simulink model "VFlexP_small"  (R2026a)
settings: Solver=ode23tb  StopTime=2  FixedStep=5e-5
values from neighbouring files (symbols this model uses):
  block_idx = evalin(mdlWks, [bvarname Generators{i} '_idx'])    [fun_init_units_callback.m]
  Fb = areas    [fun_MATPOWER_to_Excel.m]
  Fi = evalin('base', get_param(block, 'Fi'))    [fun_init_GFr.m]    (also in fun_init_intconv_DC_VSM.m)
  Lf = evalin('base', get_param(block, 'Lf'))    [fun_init_GFr.m]    (also in fun_init_intconv_DC_VSM.m)
  Rf = evalin('base', get_param(block, 'Rf'))    [fun_init_GFr.m]    (also in fun_init_intconv_DC_VSM.m)
symbols that are objects in the model workspace (value not decoded): Grid_DCop_DC_PES, Grid_DCop_DCBUCK, Grid_op_CCVSC, Grid_op_IG, Grid_op_SG, Grid_op_VSM, Grid_opDC_CCVSC, Grid_opDC_VSM, Grid_opGFr, Grid_opVCVSC
undefined symbols (not defined in the file or in its folder): block_buses_DC, CCVSC_idx, Cf, costs, costs2, DFIGs_nodes, DiscIntNeverNeededParam, entity, From_nodes, grid_linsys, Grid_op_DFIG, Grid_op_DFIG_PQ, Grid_op_MSG, Grid_op_SC, Grid_op_VCVSC, Hv, initial_states_grid, Kic, Kiv, Kp_theta, Kp_w, Kpc, Kpv, last_send, Lc, m, Matrix_flux_to_i, mD, mp, MSGs_buses, Nbuses_DC, nq, op_VCVSC, Psche, Rc, rkq1, rkq2, SCs_buses, SCs_nodes, sec_control_structure, set_asked, set_DG_up, set_extra_satur, set_sending_cost, SGs_buses, SGs_nodes, Tf, To_nodes, VI_L, VI_R, WOF_Tf, xkq1, xkq2
libraries: simulink x1045, eeGeneralControl x12, eeTransforms x1, sl_discontinuities x1
(part 1 of 50)
settings Model: Creator=atomas  LastModifiedBy=atomas
settings SolverCC: ZeroCrossControl=DisableAll
settings DataIOCC: InitialState=getstatestruct(op1)  SaveFormat=StructureWithTime
settings DebuggingCC: ReadBeforeWriteMsg=DisableAll  WriteAfterWriteMsg=DisableAll  WriteAfterReadMsg=DisableAll  MultiTaskDSMMsg=none  UnderSpecifiedDimensionMsg=warning
settings SFSimCC: SFSimEcho=off
settings SimscapeCC: SimscapeNominalValues="[{\"value\":\"1\",\"unit\":\"A\"},{\"value\":\"1\",\"unit\":\"bar\"},{\"value\":\"1\",\"unit\":\"cm^2\"},{\"value\":\"1\",\"unit\":\"cm^3/s\"},{\"value\":\"1\",\"unit\":\"kJ/kg\"},{\"value\":\"1\",\"unit\":\"kW\"},{\"value\":\"1\",\"unit\":\"l\"},{\"value\":\"1\",\"unit\":\"N\"},{\"value\":\"1\",\"unit\":\"N*m\"},{\"value\":\"1\",\"unit\":\"V\"}]"  SimscapeLogType=none  SimscapeLogDataHistory=5000.0

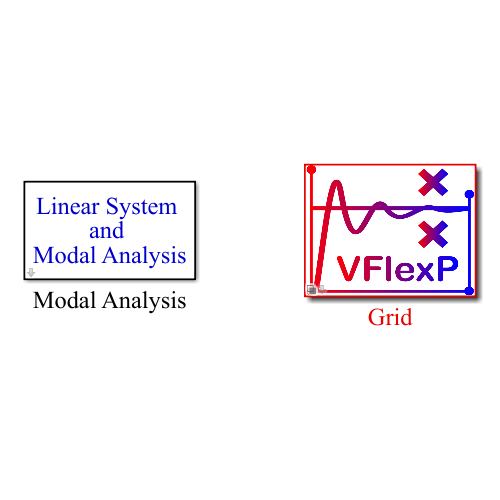
[thumbnail: Simulink's stored preview of the top-level diagram]
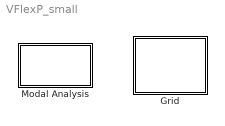
== system VFlexP_small ==
  Grid : Subsystem  Variant=on  VariantControlMode=label  VariantControl=Choice  LabelModeActiveChoice=Dynamic  mask(Grid){bvarname=Grid_, Sb=0.015, Fb_data={ '1', '50' }, bus_data={ '1', '3', '0.005', '0', '0.0001', '0.0001', '1', '1.0000000000', '0.0000000000', '230', '1', '1.1', '0.9', 'dynamic', 'series RL static omega', 'dynamic', 'PQ'; '2', '1', '0.005', '0', '0.0001', '0.0001', '1', '1.0000000000', '-0.0435875362', '230', '1', '1.1', '0.9', 'dynamic', 'series RL static omega', 'dynamic', 'PQ'; '3', '1', '0', '0', '0.0001', '0', '2', '1.0000000000', '0.6174487396', '230', '1', '1.1', '0.9', 'DC dynamic', 'DC ConstR', 'dynamic', 'PQ' }, gen_data={ '1', 'GFr', '0.0053259727', '-0.0001225105', '1000', '-1000', '1', '100', '1', '1000', '-100', '0', '0', '0', '0', '0', '0', '0', '0', '0', '0', '0'; '3', 'DC_PES', '0.0050000000', '0.0000000000', '1000', '-1000', '1', '100', '1', '1000', '-100', '0', '0', '0', '0', '0', '0', '0', '0', '0', '0', '0' }, line_data={ '1', '2', '0.005', '0.05', '0', '0', '0', '0', '0', '0', '1', '-360', '360', 'dynamic', 'static omega' }, save_in_workspace=off, parameter_change_filename=1, param_change_data={}, SC_structure=No SC, define_SC_in_MATLAB=on, delayM=0, passM=1, A_f_sc=1, A_P_sc=1, A_v_sc=1, A_Q_sc=1, g_f_sc=1, g_P_sc=1, g_v_sc=1, g_Q_sc=1, intconv_data={ 'DC_VSM', '3', '2', '0.0003', '0.0355', '0', '1000', '1000', '1000', '1', '0', '1', '-360', '360', '0', '0', '0', '0', '0', '0', '0', '0', '1', '1', '1.22', '0.75', '1', '0', '1', '-0.5', '0.5', '-360', '360', '0', '0.001', '0.0015', '0.002', '0' }, TC_structure=No TC}
      mask prompts: Sb "Base power (MW)"; Fb_data "Base frequency (Hz)"; save_in_workspace "Save in Workspace"; parameter_change_filename "Filename "Parameter_Change_V_""; SC_structure "Secondary control structure"; define_SC_in_MATLAB "Define control structure in MATLAB"; TC_structure "Tertiary control structure"
      mask init:
      | bvarname = [matlab.lang.makeValidName(get_param(gcb, 'Name')) '_'];
      |     set_param(gcb, "bvarname", bvarname)
      |     mdlWks = get_param(bdroot,'ModelWorkspace'); % Get the model workspace
      | 
      |     % Initialise variables
      |     v_buses_mod = [];
      |     Cbuses = [];
      |     DGs = [];
      |     From_buses = [];
      |     L_Lines = [];
      |     shift_lines = [];
      |     tap_lines = [];
      |     L_Loads = [];
      |     Load_buses = [];
      |     Nbuses = [];
      |     PQ_gen = [];
      |     Ploads = [];
      |     Ps_lf = [];
      |     Qloads = [];
      |     Qs_lf = [];
      |     R_Lines = [];
      |     C_Lines = [];
      |     R_Loads = [];
      |     Rcf = [];
      |     To_buses = [];
      |     Lines_fromM = [];
      |     Lines_toM = [];
      |     iPs_lf = [];
      |     iQs_lf = [];
      |     bus = [];
      |     buses_lf = [];
      |     line_complexity = [];
      |     bus_complexity = [];
      |     load_complexity = [];
      |     line_complexity_PF = [];
      |     bus_complexity_PF = [];
      |     load_complexity_PF = [];
      |     admitt_matrix = [];
      |     iadmitt_matrix = [];
      |     admitt_matrix_noloads = [];
      |     iadmitt_matrix_noloads = [];
      |     gen_static_params = [];
      |     gen_to_plot = 1;
      |     loadDC_complexity = [];
      |     lineDC_complexity = [];
      |     busDC_complexity = [];
      |     loadDC_complexity_PF = [];
      |     lineDC_complexity_PF = [];
      |     busDC_complexity_PF = [];
      |     fref.ref_units = 1;
      |     omega_base = 2*pi*50;
      | 
      |     bl = find_system([gcb '/Dynamic/Generators'], ...
      |         'IncludeCommented', 'on', 'SearchDepth', '2', ...
      |         'LookUnderMasks', 'on', 'Name', 'trim_output');
      |     for i = 1:length(bl) 
      |        DG_namei = get_param(get_param(bl{i}, 'Parent'), 'Name');
      |        eval([DG_namei 's = [];']);
      |        eval([DG_namei 's_buses = 1;']);
      |        eval([DG_namei '_idx = [];']);
      |     end
      | 
      |     try
      |         v_buses_mod = mdlWks.getVariable([bvarname 'v_buses_mod']);
      |         Cbuses = mdlWks.getVariable([bvarname 'Cbuses']);
      |         DGs = mdlWks.getVariable([bvarname 'DGs']);
      |         gen_static_params = mdlWks.getVariable([bvarname 'gen_static_params']);
      |         From_buses = mdlWks.getVariable([bvarname 'From_buses']);
      |         L_Lines = mdlWks.getVariable([bvarname 'L_Lines']);
      |         tap_lines = mdlWks.getVariable([bvarname 'tap_lines']);
      |         shift_lines = mdlWks.getVariable([bvarname 'shift_lines']);
      |         L_Loads = mdlWks.getVariable([bvarname 'L_Loads']);
      |         Load_buses = mdlWks.getVariable([bvarname 'Load_buses']);
      |         Load_busesDC = mdlWks.getVariable([bvarname 'Load_busesDC']);
      |         Nbuses = mdlWks.getVariable([bvarname 'Nbuses']);
      |         PQ_gen = mdlWks.getVariable([bvarname 'PQ_gen']);
      |         Ploads = mdlWks.getVariable([bvarname 'Ploads']);
      |         Ps_lf = mdlWks.getVariable([bvarname 'Ps_lf']);
      |         Qloads = mdlWks.getVariable([bvarname 'Qloads']);
      |         Qs_lf = mdlWks.getVariable([bvarname 'Qs_lf']);
      |         R_Lines = mdlWks.getVariable([bvarname 'R_Lines']);
      |         C_Lines = mdlWks.getVariable([bvarname 'C_Lines']);
      |         R_Loads = mdlWks.getVariable([bvarname 'R_Loads']);
      |         Rcf = mdlWks.getVariable([bvarname 'Rcf']);
      |         To_buses = mdlWks.getVariable([bvarname 'To_buses']);
      |         Lines_fromM = mdlWks.getVariable([bvarname 'Lines_fromM']);
      |         Lines_toM = mdlWks.getVariable([bvarname 'Lines_toM']);
      |         iPs_lf = mdlWks.getVariable([bvarname 'iPs_lf']);
      |         iQs_lf = mdlWks.getVariable([bvarname 'iQs_lf']);
      |         bus = mdlWks.getVariable([bvarname 'bus']);
      |         buses_lf = mdlWks.getVariable([bvarname 'buses_lf']);
      |         PloadsDC = mdlWks.getVariable([bvarname 'PloadsDC']);
      |         R_Loads_DC = mdlWks.getVariable([bvarname 'R_Loads_DC']);
      |         line_complexity = mdlWks.getVariable([bvarname 'line_complexity']);
      |         bus_complexity = mdlWks.getVariable([bvarname 'bus_complexity']);
      |         load_complexity = mdlWks.getVariable([bvarname 'load_complexity']);
      |         line_complexity_PF = mdlWks.getVariable([bvarname 'line_complexity_PF']);
      |         bus_complexity_PF = mdlWks.getVariable([bvarname 'bus_complexity_PF']);
      |         load_complexity_PF = mdlWks.getVariable([bvarname 'load_complexity_PF']);
      |         admitt_matrix = mdlWks.getVariable([bvarname 'admitt_matrix']);
      |         iadmitt_matrix = mdlWks.getVariable([bvarname 'iadmitt_matrix']);
      |         admitt_matrix_noloads = mdlWks.getVariable([bvarname 'admitt_matrix_noloads']);
      |         iadmitt_matrix_noloads = mdlWks.getVariable([bvarname 'iadmitt_matrix_noloads']);
      |         conductance_matrix = mdlWks.getVariable([bvarname 'conductance_matrix']);
      |         iconductance_matrix = mdlWks.getVariable([bvarname 'iconductance_matrix']);
      |         conductance_matrix_noloads = mdlWks.getVariable([bvarname 'conductance_matrix_noloads']);
      |         iconductance_matrix_noloads = mdlWks.getVariable([bvarname 'iconductance_matrix_noloads']);
      |         loadDC_complexity = mdlWks.getVariable([bvarname 'loadDC_complexity']);
      |         loadDC_complexity_PF = mdlWks.getVariable([bvarname 'loadDC_complexity_PF']);
      |         lineDC_complexity = mdlWks.getVariable([bvarname 'lineDC_complexity']);
      |         lineDC_complexity_PF = mdlWks.getVariable([bvarname 'lineDC_complexity_PF']);
      |         busDC_complexity = mdlWks.getVariable([bvarname 'busDC_complexity']);
      |         busDC_complexity_PF = mdlWks.getVariable([bvarname 'busDC_complexity_PF']);
      |         
      |         
      |         if length(buses_lf) <= 25
      |             gen_to_plot = 1:length(buses_lf);
      |         end
      |         for i = 1:length(bl)
      |            try
      |                DG_namei = get_param(get_param(bl{i}, 'Parent'), 'Name');
      |                aux1 = mdlWks.getVariable([bvarname DG_namei 's']);
      |                aux2 = mdlWks.getVariable([bvarname DG_namei 's_buses']);
      |                aux4 = mdlWks.getVariable([bvarname DG_namei '_idx']);
      |                eval([DG_namei 's = aux1;']);
      |                eval([DG_namei 's_buses = aux2;']);
      |                eval([DG_namei '_idx = aux4;']);
      |            catch
      |            end
      |         end
      |     if strcmp(get_param(gcb, "LabelModeActiveChoice"), "Dynamic") ...
      |                 && (strcmp(get_param([gcb '/Dynamic/Secondary Control'], ...
      |                 "LabelModeActiveChoice"), "Matrices")...
      |                 || strcmp(get_param([gcb '/Dynamic/Secondary Control'], ...
      |                 "LabelModeActiveChoice"), "Matrices1")...
      |                 || strcmp(get_param([gcb '/Dynamic/Secondary Control'], ...
      |                 "LabelModeActiveChoice"), "Matrices with delay")) ...
      |                 && ~define_SC_in_MATLAB
      |         DGs_number = length(buses_lf);
      |         delayM = 0.1*circshift(eye(DGs_number), 1);
      |         passM = circshift(eye(DGs_number), 1);
      |         A_f_sc = circshift(eye(DGs_number), 1);
      |         A_P_sc = circshift(eye(DGs_number), 1);
      |         A_v_sc = eye(DGs_number);
      |         A_Q_sc = circshift(eye(DGs_number), 1);
      |         A_f_sc(1,:) = 0;
      |         A_P_sc(1,:) = 0;
      |         A_v_sc(1,:) = 0;
      |         A_Q_sc(1,:) = 0;
      |         A_f_sc(1,1) = 0; % Leader follows reference frequency
      |         A_P_sc(1,1) = 1; % Leader is slack
      |         A_Q_sc(1,1) = 1; % Leader is slack
      |         g_f_sc = zeros(1, DGs_number);
      |         g_P_sc = zeros(1, DGs_number);
      |         g_v_sc = zeros(1, DGs_number);
      |         g_Q_sc = zeros(1, DGs_number);
      |         g_f_sc(1) = 1; % Leader follows reference frequency
      |         g_v_sc(1) = 1; % Leader follows reference voltage
      |     elseif strcmp(get_param(gcb, "LabelModeActiveChoice"), "Dynamic") ...
      |                 && strcmp(get_param([gcb '/Dynamic/Secondary Control'], ...
      |                 "LabelModeActiveChoice"), ...
      |                 "Matrices with delay and limitation") && ~define_SC_in_MATLAB
      |         DGs_number = length(buses_lf);
      |         delayM = 0*0.1*circshift(eye(DGs_number), 1);
      |         passM = circshift(eye(DGs_number), 1);
      |         A_f_sc = circshift(eye(DGs_number), 1);
      |         A_P_sc = circshift(eye(DGs_number), 1);
      |         A_v_sc = circshift(eye(DGs_number), 1);
      |         A_Q_sc = circshift(eye(DGs_number), 1);
      |         g_f_sc = zeros(1, DGs_number);
      |         g_P_sc = zeros(1, DGs_number);
      |         g_v_sc = zeros(1, DGs_number);
      |         g_Q_sc = zeros(1, DGs_number);
      |         g_f_sc(1) = 1; % Leader follows reference frequency
      |         g_v_sc(1) = 1; % Leader follows reference voltage
      |     end
      | 
      |     catch ME
      |         %errordlg(ME.message)
      |     end
      |     try
      |         DC = mdlWks.getVariable([bvarname 'DC']);
      |         intconv_PF = mdlWks.getVariable([bvarname 'intconv_PF']);
      |         fref = mdlWks.getVariable([bvarname 'fref']);
      |         omega_base = 2*pi*cell2mat(Fb_data(:,2))';
      |     catch ME
      |         %errordlg(ME.message)
      |     end
      mask Help: web('doc_Home.html')
      mask Callback bus_data: fun_bus_data_callback(gcb)
      mask Callback gen_data: fun_gen_data_callback(gcb)
      mask Callback line_data: fun_line_data_callback(gcb)
      mask Callback param_change_data: fun_apply_changes_block(gcb)
      mask TypeOptions SC_structure: No SC | Pilot nodes | Matrices | Matrices1 | Matrices with delay | Matrices with delay and limitation | MAS UC | MAS UC binary | MAS messages
      mask Callback SC_structure:
      | set_param([gcb '/Dynamic/Secondary Control'],...
      |     'LabelModeActiveChoice', ...
      |     get_param(gcb, "SC_structure"))
      mask Callback define_SC_in_MATLAB:
      | p = Simulink.Mask.get(gcb); param = p.getDialogControl('tSC_table');
      | if strcmp(get_param(gcb, "define_SC_in_MATLAB"), 'off')
      |     param.Visible = 'off';
      | else
      |     param.Visible = 'on';
      | end
      mask Callback intconv_data: fun_intconv_data_callback(gcb)
      mask TypeOptions TC_structure: No TC | MAS edp | MAS messages | Scheduled
      mask Callback TC_structure:
      | set_param([gcb '/Dynamic/Tertiary Control'],...
      |     'LabelModeActiveChoice', ...
      |     get_param(gcb, "TC_structure"))
      mask DialogControl load_system Prompt: Load system
      mask DialogControl load_system Callback: fun_load_system_callback(gcb)
      mask DialogControl save_table Prompt: Save table file
      mask DialogControl save_table Callback: fun_save_table_callback(gcb)
      mask DialogControl MATPOWER_loadflow Prompt: MATPOWER Loadflow
      mask DialogControl MATPOWER_loadflow Callback: fun_MATPOWER_loadflow(gcb)
      mask DialogControl loadflow Prompt: Loadflow
      mask DialogControl loadflow Callback: fun_loadflow_callback(gcb)
      mask DialogControl lf_report Prompt: Loadflow report
      mask DialogControl lf_report Callback: fun_lf_report_callback(gcb)
      mask DialogControl init_units Prompt: Initialise units
      mask DialogControl init_units Callback: fun_init_units_callback(gcb)
      mask DialogControl load_complexity Prompt: Load complexity in grid
      mask DialogControl load_complexity Callback: fun_load_complexity_grid(gcb)
      mask DialogControl Scope_gen Prompt: Show generators signals
      mask DialogControl Scope_gen Callback: open_system([gcb '/Dynamic/Scope_gen'])
      mask DialogControl simulate_simulink Prompt: Simulate
      mask DialogControl simulate_simulink Callback:
      | model = bdroot;
      | sim(model);
      mask DialogControl Control34 Prompt: Instituto de Investigación Tecnológica. <br> Universidad Pontificia Comillas.
      mask DialogControl Control34 Callback: web('https://www.iit.comillas.edu/')
      mask DialogControl home_tab Prompt: System parameters
      mask DialogControl new_row_Fb Prompt: +
      mask DialogControl new_row_Fb Callback: fun_mask_new_row_Fb(gcb)
      mask DialogControl delete_row_Fb Prompt: -
      mask DialogControl delete_row_Fb Callback: fun_mask_delete_row_Fb(gcb)
      mask DialogControl clear_Fb_table Prompt: Clear
      mask DialogControl clear_Fb_table Callback:
      | maskObj = Simulink.Mask.get(gcb);
      |     tableControl = maskObj.getDialogControl( 'Fb_data' );
      |     for i=1:tableControl.getNumberOfRows()
      |         tableControl.removeRow(1);
      |     end
      mask DialogControl bus_tab Prompt: Bus data
      mask DialogControl new_row_bus Prompt: +
      mask DialogControl new_row_bus Callback: fun_mask_new_row_Bus(gcb)
      mask DialogControl delete_row_bus Prompt: -
      mask DialogControl delete_row_bus Callback: fun_mask_delete_row_Bus(gcb)
      mask DialogControl clear_bus_table Prompt: Clear
      mask DialogControl clear_bus_table Callback:
      | maskObj = Simulink.Mask.get(gcb);
      |     tableControl = maskObj.getDialogControl( 'bus_data' );
      |     for i=1:tableControl.getNumberOfRows()
      |         tableControl.removeRow(1);
      |     end
      mask DialogControl gen_tab Prompt: Gen data
      mask DialogControl refresh_DGs Prompt: Refresh DG options
      mask DialogControl refresh_DGs Callback: fun_refresh_DGs_callback(gcb)
      mask DialogControl open_DG Prompt: Open DGs configuration
      mask DialogControl open_DG Callback: fun_open_DG_callback(gcb)
      mask DialogControl new_row_gen Prompt: +
      mask DialogControl new_row_gen Callback: fun_mask_new_row_Gen(gcb)
      mask DialogControl delete_row_gen Prompt: -
      mask DialogControl delete_row_gen Callback: fun_mask_delete_row_Gen(gcb)
      mask DialogControl clear_gen_table Prompt: Clear
      mask DialogControl clear_gen_table Callback:
      | maskObj = Simulink.Mask.get(gcb);
      |     tableControl = maskObj.getDialogControl( 'gen_data' );
      |     for i=1:tableControl.getNumberOfRows()
      |         tableControl.removeRow(1);
      |     end
      mask DialogControl line_tab Prompt: Line data
      mask DialogControl new_row_line Prompt: +
      mask DialogControl new_row_line Callback: fun_mask_new_row_Line(gcb)
      mask DialogControl delete_row_line Prompt: -
      mask DialogControl delete_row_line Callback: fun_mask_delete_row_Line(gcb)
      mask DialogControl clear_line_table Prompt: Clear
      mask DialogControl clear_line_table Callback:
      | maskObj = Simulink.Mask.get(gcb);
      |     tableControl = maskObj.getDialogControl( 'line_data' );
      |     for i=1:tableControl.getNumberOfRows()
      |         tableControl.removeRow(1);
      |     end
      mask DialogControl param_change Prompt: Parameter Variation
      mask DialogControl execute_parameter_change Prompt: Execute Parameter Change
      mask DialogControl execute_parameter_change Callback: fun_execute_parameter_change(gcb)
      mask DialogControl new_parameter Prompt: +
      mask DialogControl new_parameter Callback: fun_mask_new_row_Param(gcb)
      mask DialogControl delete_parameter Prompt: -
      mask DialogControl delete_parameter Callback: fun_mask_delete_row_Param(gcb)
      mask DialogControl clear_param_table Prompt: Clear
      mask DialogControl clear_param_table Callback:
      | maskObj = Simulink.Mask.get(gcb);
      |     tableControl = maskObj.getDialogControl( 'param_change_data' );
      |     for i=1:tableControl.getNumberOfRows()
      |         tableControl.removeRow(1);
      |     end
      mask DialogControl plot_change_parameter Prompt: Plot Selected Parameter
      mask DialogControl plot_change_parameter Callback: fun_plot_change_parameter_callback(gcb)
      mask DialogControl Secondary_control Prompt: Secondary control
      mask DialogControl Construct_MAS Prompt: Construct_MAS
      mask DialogControl Construct_MAS Callback: fun_construct_MAS_callback(gcb)
      mask DialogControl Initialise_0 Prompt: Initialise all variables to 0
      mask DialogControl Initialise_0 Callback: fun_initialise_0_callback(gcb)
      mask DialogControl intconv_tab Prompt: Int converters
      mask DialogControl new_row_intconv Prompt: +
      mask DialogControl new_row_intconv Callback: fun_mask_new_row_Intconv(gcb)
      mask DialogControl delete_row_intconv Prompt: -
      mask DialogControl delete_row_intconv Callback: fun_mask_delete_row_Intconv(gcb)
      mask DialogControl clear_intconv_tabl Prompt: Clear
      mask DialogControl clear_intconv_tabl Callback:
      | maskObj = Simulink.Mask.get(gcb);
      |     tableControl = maskObj.getDialogControl( 'intconv_data' );
      |     for i=1:tableControl.getNumberOfRows()
      |         tableControl.removeRow(1);
      |     end
      mask DialogControl Tertiary_control Prompt: Tertiary control
      mask DialogControl Construct_MAS_tertiary Prompt: Construct_MAS
      mask DialogControl Construct_MAS_tertiary Callback: fun_construct_MAS_callback(gcb)
      mask DialogControl Initialise_0_copy Prompt: Initialise all variables to 0
      mask DialogControl Initialise_0_copy Callback: fun_initialise_0_callback(gcb)
      mask Display: image('$imagefile');
  Modal Analysis : Subsystem
      mask Help: web([extractBefore(get_param(bdroot, 'FileName'), ['\' gcs '.slx']) '\Documentation\modal_analysis.html'])
      mask DialogControl DescTextVar Prompt: FAST MODAL ANALYSIS TOOL
      mask DialogControl ParameterGroupVar Prompt: ANALYSIS
      mask DialogControl calculate_linsys Prompt: Calculate Linear System
      mask DialogControl calculate_linsys Callback:
      | wb = waitbar(0, 'Linearizing the system', 'Name','Linear System Option'); % Waitbar
      |     model = bdroot;
      |     io = getlinio(model);
      |     waitbar(0.25,wb)
      |     try
      |         linsys = linearize(model,io);
      |          waitbar(0.5,wb)
      |         if height(linsys)>1
      |             linsys = linsys(1,1);
      |         end
      |             waitbar(0.75,wb)
      |         modelworkspace=get_param(model,"ModelWorkspace");
      | 
      |         assignin("base","linsys",linsys);
      |         assignin(modelworkspace,"linsys",linsys);
      |         waitbar(1,wb)
      | 
      |     catch
      |         try
      |         waitbar(0.5,wb)
      |         linsys = linearize(model,io);
      |         waitbar(0.75,wb)
      |         if height(linsys)>1
      |             linsys = linsys(1,1);
      |         end
      |         waitbar(1,wb)
      |         modelworkspace=get_param(model,"ModelWorkspace");
      | 
      |         assignin("base","linsys",linsys);
      |         assignin(modelworkspace,"linsys",linsys);
      |         catch ME
      |              msg = ["There has being a problem calculating the modal analysis",...
      |             "Please check:"," - (1) you are working on the simulink model folder",...
      |             " - (2) The scripts for the linearized trigonometric functions are " + ...
      |             "in the same folder",...
      |             " - (3) There is still one input perturbation and one output measurement in the system"];
      |             errordlg(msg);
      |             errordlg(ME.message);
      |         end
      |     end
      | 
      |     close(wb)
      mask DialogControl modal_analysis_calculation Prompt: Modal Analysis Excel Generator
      mask DialogControl modal_analysis_calculation Callback:
      | wb = waitbar(0, 'Modal Analisys', 'Name','Exporting Modal Analysis Caculation'); % Waitbar
      | 
      |     model = bdroot;
      |     waitbar(0.25,wb)
      |     modelworkspace=get_param(model,"ModelWorkspace");
      |     linsys = evalin(modelworkspace,"linsys");
      |   if ~isempty(linsys)
      |         A = linsys.a;
      |       [v,z] = eig(A);
      |         n = height(A);
      |         % Eigenvalues
      |         z = diag(z) ;
      |         %[magz,iz]=sort(1./abs(z));
      |         [~,iz]=sort(1./imag(z));
      |         z = z(iz);
      |         v = v(:,iz);
      |         % Right eigenvectors
      |         for i = 1:n
      |           [~,imax] = max(abs(v(:,i))) ;
      |           v(:,i) = v(:,i)/v(imax,i) ;
      |         end
      |         % Left eigenvectors
      |         w=inv(v);
      |         % Participations
      |         for i = 1:n
      |           for j = 1:n
      |             p(i,j) = w(j,i)*v(i,j);
      |           end
      |         end
      |                 Xvec_vars = linsys.StateName;
      | 
      |     waitbar(0.5,wb)
      | 
      |     N = height(A);
      |     nombrevar = char(Xvec_vars);
      | 
      |     Variables_Names = char(nombrevar);
      |     Modes = string(1:N)';
      |     T1 = table(Variables_Names);
      |     T =  array2table(abs(p));
      |     T.Properties.VariableNames = Modes;
      |     TPart = [T1 T];
      |     waitbar(0.6,wb)
      | 
      |     TeigenvaluesTitle = ({'Eigenvalue'; 'REAL';'IMAGINARY';'DAMPING';'FREQUENCY'});
      |     Eig_Table = [ array2table([ (1:length(z))' real(z) imag(z) -real(z)./abs(z)*100,abs(z)./2/pi])];
      |     Eig_Table.Properties.VariableNames = TeigenvaluesTitle;
      |     waitbar(0.7,wb)
      | 
      |     unstable_eigenvalues = find(real(z)>0);
      | 
      |      if unstable_eigenvalues>1
      |         TPart_Unstable = sortrows([T1 TPart(:,unstable_eigenvalues+1)],2,{'descend'});
      |      end
      |     else
      |         msg = "There has being a problem calculating the modal analysis";
      |         f = warndlg(msg);
      |     end
      |     try
      |         filename ="ModalAnalysisTables.xlsx";
      |         writetable(sortrows(Eig_Table,4,{'ascend'}),filename,"Sheet","SUMMARY BY DAMPING");
      |         writetable(sortrows(Eig_Table,5,{'ascend'}),filename,"Sheet","SUMMARY BY FREQUENCY");
      |     waitbar(0.8,wb)
      | 
      |         writetable(TPart,filename,"Sheet","Participations");
      |         if (unstable_eigenvalues)>1
      |             writetable(TPart_Unstable,filename,"Sheet","Unstable Participations");
      |         else
      |             writematrix([0 0],filename,"Sheet","Unstable Participations");
      |         end
      |         writematrix([real(v) imag(v)],filename,"Sheet","Left Eigenvectors");
      |         waitbar(0.9,wb)
      | 
      |         writematrix([real(w) imag(w)],filename,"Sheet","Right Eigenvectors");
      |         waitbar(1,wb)
      | 
      |         msg = "TABLES HAVE BEEN CORRECTLY EXPORTED";
      |         f = warndlg(msg);
      |     catch
      |          msg = ["TABLES COULD NOT BE MADE"," MAKE SURE THE EXCEL IS CLOSED"];
      |          f = warndlg(msg);
      | 
      | 
      |     end
      |         close(wb)
      mask DialogControl plot_eigenvalues Prompt: Plot EigenValues
      mask DialogControl plot_eigenvalues Callback:
      | model = bdroot;
      | 
      |     modelworkspace=get_param(model,"ModelWorkspace");
      |     linsys = evalin(modelworkspace,"linsys");
      | 
      |     figure(1);clf;
      |     plot(real(eig(linsys.a)),imag(eig(linsys.a)),'*');
      |     grid on
      mask DialogControl plot_eigenvalues_mod_angle Prompt: Plot Eigenvalues Mod&Angle
      mask DialogControl plot_eigenvalues_mod_angle Callback:
      | model = bdroot;
      | 
      | modelworkspace=get_param(model,"ModelWorkspace");
      | linsys = evalin(modelworkspace,"linsys");
      | figure(1);clf;
      | loglog(abs(eig(linsys.a)),rad2deg(wrapTo2Pi(angle(eig(linsys.a)))),'*');
      | 
      | xlimit = log10(xlim); %ylimit = ylim;
      | 
      | for i=logspace(2*xlimit(1)-xlimit(2),xlimit(2),40)
      |     line(min(max(i./abs(cos(deg2rad(90:1:270))),0.99*10^xlimit(1)), ...
      |     1.01*10^xlimit(2)),90:1:270,'LineStyle','-','Color','black','HandleVisibility','off');
      | end
      | 
      | ylim([90-20 180])
      mask DialogControl run_andres_tool Prompt: Advanced Simulink Modal Analysis Tool
      mask DialogControl run_andres_tool Callback: simulink_modal_analysis(bdroot);
      mask DialogControl Container3 Prompt: CLEAR SYSTEMS
      mask DialogControl clear_simulink Prompt: Clear SIMULINK Workspace
      mask DialogControl clear_simulink Callback:
      | model = bdroot;
      |     command_clear = "clear all";
      | 
      |     modelworkspace=get_param(model,"ModelWorkspace");
      |     evalin(modelworkspace,command_clear)
      mask DialogControl clear_matlab Prompt: Clear MATLAB Workspaces
      mask DialogControl clear_matlab Callback:
      | command_clear = "clear all";
      |     evalin("base",command_clear)
      mask Display:
      | color('BLUE');
      | 
      | fprintf('Linear System \nand \nModal Analysis');

== system VFlexP_small/Grid ==
  Dynamic : Subsystem  VariantControl=Dynamic
  Loadflow : Subsystem  VariantControl=Loadflow

== system VFlexP_small/Modal Analysis ==

== system VFlexP_small/Grid/Dynamic ==
  Constant2 : Constant  Value=omega_base  VectorParams1D=off
  DCAC converters : Subsystem
  Display : Display
  Display1 : Display
  Display2 : Display
  Fault : Subsystem  Commented=on
  Gain : Gain  Gain=1/(2*pi)
  Gain1 : Gain  Gain=Sb
  Gain2 : Gain  Gain=Sb
  Gain3 : Gain  Gain=Sb
  Gain4 : Gain  Gain=0.5
  Gain{5..8} (4 alike) : Gain  Gain=50
  Generators : Subsystem
  Generators_DC : Subsystem
  Goto Tag Visibility : GotoTagVisibility  GotoTag=omega_ref
  Goto Tag Visibility1 : GotoTagVisibility  GotoTag=omega_base
  Grid : Subsystem  Variant=on  VariantControlMode=label  LabelModeActiveChoice=Dynamic
  Grid_DC : Subsystem  Variant=on  VariantControlMode=label  LabelModeActiveChoice=Dynamic
  Grid_linear : Subsystem  Commented=on
  Integrator : Integrator  InitialConditionSource=external
  Integrator1 : Integrator  InitialConditionSource=external
  LPF : Subsystem
  LPF1 : Subsystem
  LPF2 : Subsystem
  LPF3 : Subsystem
  Manual Switch : ManualSwitch
  One : Constant  OutDataTypeStr=Inherit: Inherit via back propagation
  Product1 : Product
  Product2 : Product
  Real-Imag to Complex1 : RealImagToComplex
  Real-Imag to Complex2 : RealImagToComplex
  Scope{,2..4} (4 alike) : Scope
      Scope settings: ActiveDisplayYMinimum=0.0022712  ActiveDisplayYMaximum=0.0044108
      Scope2 settings: ActiveDisplayYMinimum=49.851  ActiveDisplayYMaximum=50.0166  DataLoggingVariableName=ScopeData11
      Scope3 settings: ActiveDisplayYMinimum=49.8343  ActiveDisplayYMaximum=50.0185  DataLoggingVariableName=ScopeData12
      Scope4 settings: ActiveDisplayYMinimum=49.83966644890701  ActiveDisplayYMaximum=50.01785268343977
  Scope1 : Scope  NumInputPorts=2
      settings: ActiveDisplayYMinimum=-0.03276  ActiveDisplayYMaximum=0.28873  DataLoggingVariableName=ScopeData8
  Scope_gen : Scope  NumInputPorts=4
      settings: Title=Frequency (Hz)  ActiveDisplayYMinimum=49.889931736775623  ActiveDisplayYMaximum=50.01222980702493  DataLoggingVariableName=gen
  Secondary Control : Subsystem  Variant=on  VariantControlMode=label  VariantControl=Choice  LabelModeActiveChoice=No SC
      settings: PortSchema="{\"entries\":[{\"content\":{\"sides\":[{\"content\":{\"connectorIds\":[\"Out1\"]},\"type\":\"ConnectorPlacement.EquallySpacedRectSide\",\"uuid\":\"fff1731e-03ae-4532-8327-8c877d5503a1\"},{\"content\":{\"connectorIds\":[\"In1\",\"In2\",\"In3\",\"In4\"],\"side\":\"RIGHT\"},\"type\":\"ConnectorPlacement.EquallySpacedRectSide\",\"uuid\":\"a483b49e-8899-40e0-871c-863b08e1ecd3\"},{\"content\":{\"connectorIds\":[],\"side\":\"TOP\"},\"type\":\"ConnectorPlacement.EquallySpacedRectSide\",\"uuid\":\"d6acdfc2-068d-45c3-a7db-011142f68adc\"},{\"content\":{\"connectorIds\":[],\"side\":\"BOTTOM\"},\"type\":\"ConnectorPlacement.EquallySpacedRectSide\",\"uuid\":\"a007924e-be31-4ab9-87dc-62addce8969f\"}]},\"type\":\"ConnectorPlacement.EquallySpacedConnector\",\"uuid\":\"f40773b4-1769-44e6-aa19-3b4c4e232e75\"}],\"packageUris\":[\"http://schema.mathworks.com/mf0/Connector/R2020b\"],\"version\":\"1.0\"}"
  Selector : Selector  NumberOfDimensions=2  InputPortWidth=3  IndexOptions=Index vector (dialog),Index vector (dialog)  Indices=1,fref.ref_units  OutputSizes=1,1
  Selector1 : Selector  NumberOfDimensions=2  InputPortWidth=3  IndexOptions=Select all,Index vector (dialog)  Indices=[1 3],gen_to_plot  OutputSizes=1,1
  Selector10 : Selector  NumberOfDimensions=2  InputPortWidth=3  IndexOptions=Index vector (dialog),Select all  Indices=2,1  OutputSizes=1,1
  Selector11 : Selector  NumberOfDimensions=2  InputPortWidth=3  IndexOptions=Index vector (dialog),Select all  Indices=4,1  OutputSizes=1,1
  Selector2 : Selector  NumberOfDimensions=2  InputPortWidth=3  IndexOptions=Index vector (dialog),Index vector (dialog)  Indices=2,1  OutputSizes=1,1
  Selector3 : Selector  NumberOfDimensions=2  InputPortWidth=3  IndexOptions=Index vector (dialog),Select all  Indices=2,1  OutputSizes=1,1
  Selector4 : Selector  NumberOfDimensions=2  InputPortWidth=3  IndexOptions=Index vector (dialog),Index vector (dialog)  Indices=1,1  OutputSizes=1,1
  Selector5 : Selector  NumberOfDimensions=2  InputPortWidth=3  IndexOptions=Index vector (dialog),Select all  Indices=3,1  OutputSizes=1,1
  Selector7 : Selector  NumberOfDimensions=2  InputPortWidth=3  IndexOptions=Index vector (dialog),Select all  Indices=1,1  OutputSizes=1,1
  Selector8 : Selector  InputPortWidth=length(fref.ref_units)  IndexOptions=Index vector (dialog)  Indices=fref.Fb_units  OutputSizes=1
  Selector9 : Selector  NumberOfDimensions=2  InputPortWidth=3  IndexOptions=Index vector (dialog),Select all  Indices=1,1  OutputSizes=1,1
  Step : Step  Time=20  SampleTime=0  VectorParams1D=off  ZeroCross=off
  Step1 : Step  Time=10  InitialValue=ones(1, length(buses_lf))  FinalValue=[ones(1, length(buses_lf)-1) 1]  SampleTime=0  VectorParams1D=off  ZeroCross=off
  Subsystem1 : Subsystem  Commented=on
  Sum : Sum  Inputs=+++++
  Sum1 : Sum  Inputs=|++
  Sum2 : Sum  Inputs=|++
  Sum3 : Sum  Inputs=|+-
  Sum4 : Sum  Inputs=|+-
  Sum5 : Sum  Inputs=|++
  Terminator : Terminator
  Terminator1 : Terminator
  Tertiary Control : Subsystem  Variant=on  VariantControlMode=label  VariantControl=Choice  LabelModeActiveChoice=No TC
      settings: PortSchema="{\"entries\":[{\"content\":{\"sides\":[{\"content\":{\"connectorIds\":[\"Out1\"]},\"type\":\"ConnectorPlacement.EquallySpacedRectSide\",\"uuid\":\"fff1731e-03ae-4532-8327-8c877d5503a1\"},{\"content\":{\"connectorIds\":[\"In1\",\"In2\",\"In3\"],\"side\":\"RIGHT\"},\"type\":\"ConnectorPlacement.EquallySpacedRectSide\",\"uuid\":\"a483b49e-8899-40e0-871c-863b08e1ecd3\"},{\"content\":{\"connectorIds\":[],\"side\":\"TOP\"},\"type\":\"ConnectorPlacement.EquallySpacedRectSide\",\"uuid\":\"d6acdfc2-068d-45c3-a7db-011142f68adc\"},{\"content\":{\"connectorIds\":[],\"side\":\"BOTTOM\"},\"type\":\"ConnectorPlacement.EquallySpacedRectSide\",\"uuid\":\"a007924e-be31-4ab9-87dc-62addce8969f\"}]},\"type\":\"ConnectorPlacement.EquallySpacedConnector\",\"uuid\":\"f40773b4-1769-44e6-aa19-3b4c4e232e75\"}],\"packageUris\":[\"http://schema.mathworks.com/mf0/Connector/R2020b\"],\"version\":\"1.0\"}"
  To Workspace : ToWorkspace  VariableName=elec  SaveFormat=Timeseries  SampleTime=-1
  To Workspace1 : ToWorkspace  Commented=on  VariableName=v_buses_DC  SaveFormat=Timeseries  SampleTime=-1
  iP : Subsystem  Commented=on
  in_current : Subsystem
  in_current_bus : Subsystem
  mod pilot buses1 : Subsystem
  v1 : ComplexToMagnitudeAngle  Output=Magnitude
  vall : ComplexToMagnitudeAngle  Output=Magnitude
  tag scope: omega_base=scoped, omega_ref=scoped
  wires:
  Generators/1(i) -> [i_from_gen]
  [elec] -> Selector/1
  Selector3/1 -> Integrator/2, Sum3/1, LPF1/1(In1)  "P"
  Selector5/1 -> LPF2/1(In1)  "v"
  Selector11/1 -> LPF3/1(In1)  "Q"
  Secondary Control/1(secondary_refs) -> Generators/2(ref)
  Product1/1 -> Gain/1
  Gain2/1 -> Scope_gen/4  "Q"
  [v_buses] -> Generators/1(v)
  Generators/2(elec) -> To Workspace/1, [elec]
  Selector1/1 -> Selector7/1, Selector11/1, Selector5/1, Selector3/1
  [elec] -> Selector1/1
  [i_from_gen] -> Sum/2
  One/1 -> Manual Switch/2
  Grid_DC/1(v_buses_dc) -> To Workspace1/1, [v_buses_DC]
  [v_buses] -> DCAC converters/1(vac)
  [v_buses_DC] -> DCAC converters/2(vdc)
  Sum/1 -> Grid_linear/1(In1), Grid/1(i_from_gen)
  Step1/1 -> Tertiary Control/1(connect_DGs)
  [elec] -> Tertiary Control/3(elec)
  [v_buses] -> mod pilot buses1/1(v)
  mod pilot buses1/1(vmod) -> Tertiary Control/2(vmod)
  [v_buses] -> Secondary Control/4(v_buses)
  [elec] -> Secondary Control/2(elec)
  Constant2/1 -> [omega_base]
  Selector7/1 -> Gain7/1, Sum5/2, LPF/1(In1)  "f"
  [omega_base] -> Selector8/1
  Selector8/1 -> Product1/1
  Gain/1 -> Scope_gen/1  "f"
  DCAC converters/2(idc) -> Sum2/1
  Sum2/1 -> Grid_DC/1(i_from_gen_dc)
  Generators_DC/1(i) -> Product2/2, Sum2/2
  [v_buses_DC] -> Product2/1, Generators_DC/1(v)
  DCAC converters/1(iac) -> Sum/4
  Manual Switch/1 -> [omega_ref]
  Selector/1 -> Manual Switch/1
  Product2/1 -> Gain3/1
  Gain3/1 -> Scope/1
  [v_buses] -> iP/1(v)
  Gain1/1 -> Scope_gen/2  "P"
  Step/1 -> Secondary Control/1(start_SC)
  in_current/1(i) -> Sum/3
  iP/1(i) -> Sum/1
  [v_buses] -> in_current/1(v)
  Real-Imag to Complex1/1 -> vall/1
  Selector9/1 -> Real-Imag to Complex1/1
  Selector10/1 -> Real-Imag to Complex1/2
  vall/1 -> Terminator/1
  Selector2/1 -> Real-Imag to Complex2/2
  Selector4/1 -> Real-Imag to Complex2/1
  Real-Imag to Complex2/1 -> v1/1
  [v_buses] -> Selector2/1, Selector4/1, Selector10/1, Selector9/1
  v1/1 -> Terminator1/1
  in_current_bus/1(Out1) -> Sum/5
  Grid/1(v_buses) -> Sum1/1
  Sum1/1 -> [v_buses]
  Grid_linear/1(Out1) -> Sum1/2
  LPF/1(Out1) -> Product1/2
  LPF2/1(Out1) -> Scope_gen/3
  LPF3/1(Out1) -> Gain2/1
  Tertiary Control/1(ref) -> Secondary Control/3(tertiary_refs)
  Integrator/1 -> Sum3/2
  Integrator1/1 -> Sum4/2
  [Pi_VSM] -> Integrator1/2, Sum4/1
  Sum4/1 -> Scope1/2
  Sum3/1 -> Scope1/1
  LPF1/1(Out1) -> Gain1/1
  Sum5/1 -> Gain4/1
  Gain4/1 -> Gain5/1
  Gain5/1 -> Display/1, Scope2/1
  Gain6/1 -> Display1/1
  [omega_DC_VSM] -> Gain6/1, Gain8/1, Sum5/1
  Gain7/1 -> Scope3/1, Display2/1  "freq_GFor_no_limited"
  Gain8/1 -> Scope4/1

== system VFlexP_small/Grid/Loadflow ==
  Generators : Subsystem
  Goto Tag Visibility : GotoTagVisibility  GotoTag=omega_ref
  Grid : Subsystem  Variant=on  VariantControlMode=label  LabelModeActiveChoice=Dynamic
  Loads : Subsystem
  One : Constant  OutDataTypeStr=Inherit: Inherit via back propagation
  Selector2 : Selector  InputPortWidth=Nbuses  IndexOptions=Index vector (dialog)  Indices=Load_buses  OutputSizes=1
  Selector3 : Selector  InputPortWidth=Nbuses  IndexOptions=Index vector (dialog)  Indices=Load_buses  OutputSizes=1
  to_all_Nodes : Subsystem
  to_all_Nodes1 : Subsystem
  tag scope: omega_ref=scoped
  wires:
  One/1 -> [omega_ref]
  Generators/2(i_q) -> Grid/2(iq_in)
  Generators/1(i_d) -> Grid/1(id_in)
  to_all_Nodes/1(id_out) -> Grid/3(id_out)
  to_all_Nodes1/1(iq_out) -> Grid/4(iq_out)
  Loads/1(id) -> to_all_Nodes/1(In1)
  Loads/2(iq) -> to_all_Nodes1/1(In1)
  Selector2/1 -> Loads/1(vd)
  Selector3/1 -> Loads/2(vq)
  Grid/1(vd) -> Generators/1(vd), Selector2/1
  Grid/2(vq) -> Selector3/1, Generators/2(vq)
